simulink model "finalmodel6"  (Simulink 7.5)
settings: Solver=ode23t  StartTime=0.0  StopTime=5  RelTol=1e-3
undefined symbols (not defined in the file): DiscIntNeverNeededParam
libraries: powerlib x5, simulink_extras x3, dspinverses x1, simulink x1
settings Model: Creator=comp  LastModifiedBy=comp

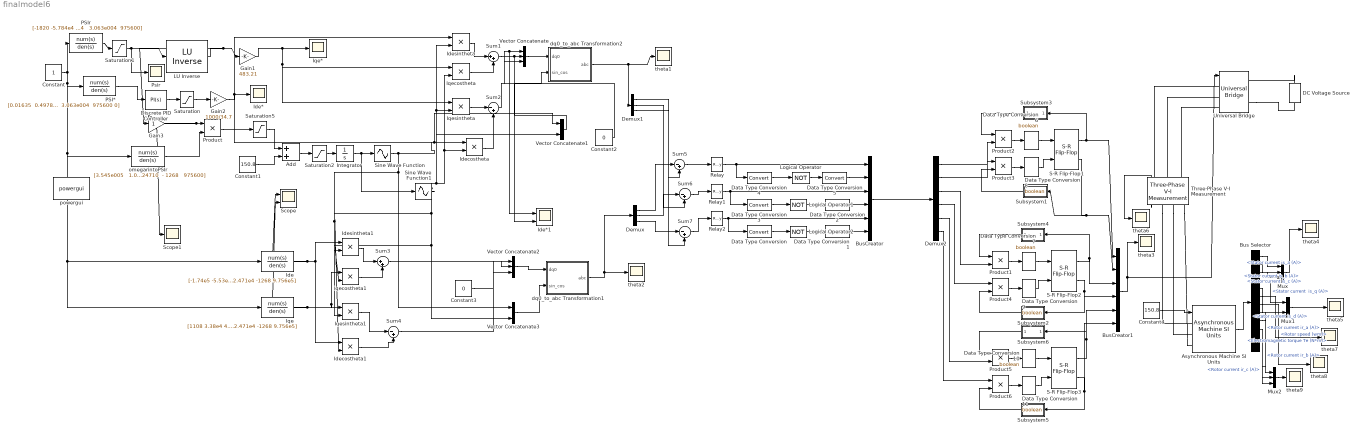
== system finalmodel6 ==
  " LU Inverse" : dspinverses/ LU Inverse  SystemSampleTime=-1
  " omegarintoPSIr" : TransferFcn  Numerator="[3.545e005   1.081e007   1.281e007  - 1.072e010]"  Denominator="[1 - 0.1335  24710  - 1268   975600]"
  Add : Sum  OutDataType=fixdt(1, 16)  OutScaling=2^-10
  Asynchronous Machine SI Units : powerlib/Machines/Asynchronous Machine SI Units  DialogController=POWERSYS.PowerSysDialog  SystemSampleTime=-1  PresetModel=No  MechanicalLoad=Speed w  ShowDetailedParameters=on  RotorType=Squirrel-cage  ReferenceFrame=Stationary  NominalParameters=[149.2e3 400 50]  Stator=[14.85e-3 .3027e-3]  Rotor=[9.295e-3 .3027e-3]  Lm=10.46e-3  Mechanical=[0.0131 0.002985 2]  PolePairs=2  InitialConditions=[1 0 0 0 0 0 0 0]  Units=SI  LoadFlowParameters=1492000  SimulateSaturation=off  Saturation=[14.03593122, 27.81365428, 53.79336849, 72.68890987, 97.98006896, 148.6815601, 215.7428561, 302.9841135, 428.7778367 ; 230, 322, 414, 460, 506, 552, 598, 644, 690]  TsPowergui=0  TsBlock=-1  IterativeModel=Forward Euler
  Bus Selector : BusSelector  OutputSignals="Stator measurements.Stator current is_a (A),Stator measurements.Stator current is_b (A),Stator measurements.Stator current is_c (A),Stator measurements.Stator current  is_q (A),Stator measurements.Stator current is_d (A),Mechanical.Electromagnetic torque Te (N*m),Mechanical.Rotor speed (wm),Rotor measurements.Rotor current ir_a (A),Rotor measurements.Rotor current ir_b (A),Rotor measurements.Rotor current ir_c (A),Rotor measurements.Rotor voltage Vr_q (V),Rotor measurements.Rotor voltage Vr_d (V)"
  BusCreator : BusCreator  Inputs=6
  BusCreator1 : BusCreator  Inputs=6
  Constant : Constant  OutDataType=fixdt(1, 16)  OutScaling=2^0
  Constant1 : Constant  Value=150.8  OutDataType=fixdt(1, 16)  OutScaling=2^0
  Constant2 : Constant  Value=0  OutDataType=fixdt(1, 16)  OutScaling=2^0
  Constant3 : Constant  Value=0  OutDataType=fixdt(1, 16)  OutScaling=2^0
  Constant4 : Constant  Value=150.8  OutDataType=fixdt(1, 16)  OutScaling=2^0
  DC Voltage Source : powerlib/Electrical Sources/DC Voltage Source  DialogController=POWERSYS.PowerSysDialog  SystemSampleTime=-1  Amplitude=400  Measurements=Voltage
  Data Type Conversion{,1..5} (6 alike) : DataTypeConversion  OutDataType=sfix(16)  OutScaling=2^0  SaturateOnIntegerOverflow=on  RndMeth=Zero
  Data Type Conversion{6..11} (6 alike) : DataTypeConversion  OutDataTypeMode=boolean  OutDataType=sfix(16)  OutScaling=2^0  OutDataTypeStr=boolean
  Demux : Demux  Outputs=3
  Demux1 : Demux  Outputs=3
  Demux2 : Demux  Outputs=6
  Discrete PID Controller : simulink/Continuous/PID Controller  DialogController=pidpack.PIDConfig.pidDDGCreate  DialogControllerArgs=DataTag0  SystemSampleTime=-1  Controller=PI  TimeDomain=Continuous-time  SampleTime=1  IntegratorMethod=Forward Euler  FilterMethod=Forward Euler  Form=Parallel  P=100  I=30  D=0  N=100  InitialConditionSource=internal  InitialConditionForIntegrator=0  InitialConditionForFilter=0  ExternalReset=none  LimitOutput=off  UpperSaturationLimit=inf  LowerSaturationLimit=-inf  LinearizeAsGain=off  AntiWindupMode=none  Kb=1  TrackingMode=off  Kt=1  PParamMin=[]  PParamMax=[]  IParamMin=[]  IParamMax=[]  DParamMin=[]  DParamMax=[]  NParamMin=[]  NParamMax=[]  KbParamMin=[]  KbParamMax=[]  KtParamMin=[]  KtParamMax=[]  POutMin=[]  POutMax=[]  IOutMin=[]  IOutMax=[]  DOutMin=[]  DOutMax=[]  NOutMin=[]  NOutMax=[]  KbOutMin=[]  KbOutMax=[]  KtOutMin=[]  KtOutMax=[]  IntegratorOutMin=[]  IntegratorOutMax=[]  FilterOutMin=[]  FilterOutMax=[]  SumOutMin=[]  SumOutMax=[]  SumI1OutMin=[]  SumI1OutMax=[]  SumI2OutMin=[]  SumI2OutMax=[]  SumI3OutMin=[]  SumI3OutMax=[]  SumDOutMin=[]  SumDOutMax=[]  SaturationOutMin=[]  SaturationOutMax=[]  IntegratorContinuousStateAttributes=''  IntegratorStateMustResolveToSignalObject=off  IntegratorRTWStateStorageClass=Auto  FilterContinuousStateAttributes=''  FilterStateMustResolveToSignalObject=off  FilterRTWStateStorageClass=Auto
  Gain1 : Gain  Gain=483.21  ParameterDataType=fixdt(1, 16)  ParameterScaling=2^0  OutDataType=fixdt(1, 16)  OutScaling=2^0  SampleTime=5e-5
  Gain2 : Gain  Gain=1000/34.7  ParameterDataType=fixdt(1, 16)  ParameterScaling=2^0  OutDataType=fixdt(1, 16)  OutScaling=2^0  SampleTime=5e-5
  Gain3 : Gain  ParameterDataType=fixdt(1, 16)  ParameterScaling=2^0  OutDataType=fixdt(1, 16)  OutScaling=2^0  SampleTime=5e-5
  Ide : TransferFcn  Numerator=[-1.74e5 -5.53e6 -6.725e6]  Denominator=[1 -.1335 2.471e4 -1268 9.756e5]
  Ide* : Scope
      settings: YMin=-100  YMax=100
  Ide*1 : Scope  NumInputPorts=2
      settings: YMin=-10000~-1000  YMax=10000~1000  SaveName=ScopeData5
  Idecostheta : Product  OutDataType=fixdt(1, 16)  OutScaling=2^0  RndMeth=Zero
  Idecostheta1 : Product  OutDataType=fixdt(1, 16)  OutScaling=2^0  RndMeth=Zero
  Idesintheta : Product  OutDataType=fixdt(1, 16)  OutScaling=2^0  RndMeth=Zero
  Idesintheta1 : Product  OutDataType=fixdt(1, 16)  OutScaling=2^0  RndMeth=Zero
  Integrator : Integrator  UpperSaturationLimit=pi/5  LowerSaturationLimit=0
  Iqe : TransferFcn  Numerator=[1108 3.38e4 4.003e4 -3.349e7]  Denominator=[1 -.1335 2.471e4 -1268 9.756e5]
  Iqe* : Scope
      settings: YMin=-200  YMax=200
  Iqecostheta : Product  OutDataType=fixdt(1, 16)  OutScaling=2^0  RndMeth=Zero
  Iqecostheta1 : Product  OutDataType=fixdt(1, 16)  OutScaling=2^0  RndMeth=Zero
  Iqesintheta : Product  OutDataType=fixdt(1, 16)  OutScaling=2^0  RndMeth=Zero
  Iqesintheta1 : Product  OutDataType=fixdt(1, 16)  OutScaling=2^0  RndMeth=Zero
  Logical Operator : Logic  Operator=NOT
  Logical Operator1 : Logic  Operator=NOT
  Logical Operator2 : Logic  Operator=NOT
  Mux : Mux  Inputs=3
  Mux1 : Mux  Inputs=2
  Mux2 : Mux  Inputs=3
  PSI* : TransferFcn  Numerator="[0.01635  0.4978 2224  7.018e004  8.566e004   487800]"  Denominator="[0.03269 0.9956  807.7  2.467e004  3.063e004  975600 0]"
  PSIr : TransferFcn  Numerator=[-1820 -5.784e4 -7.034e4]  Denominator="[0.03269   0.9956   807.7   2.467e004   3.063e004  975600]"
  Product : Product  OutDataType=fixdt(1, 16)  OutScaling=2^0  RndMeth=Zero
  Product{1..6} (6 alike) : Product  OutDataType=sfix(16)  OutScaling=2^0  RndMeth=Zero
  Psir : Scope
      settings: YMin=-10  YMax=10  SaveName=ScopeData4
  Relay : Relay  OnSwitchValue=5  OffSwitchValue=-5  OutDataType=sfix(16)  OutScaling=2^0
  Relay1 : Relay  OnSwitchValue=5  OffSwitchValue=-5  OutDataType=sfix(16)  OutScaling=2^0
  Relay2 : Relay  OnSwitchValue=5  OffSwitchValue=-5  OutDataType=sfix(16)  OutScaling=2^0
  S-R Flip-Flop1 : simulink_extras/Flip Flops/S-R Flip-Flop  SystemSampleTime=-1  initial_condition=0
  S-R Flip-Flop2 : simulink_extras/Flip Flops/S-R Flip-Flop  SystemSampleTime=-1  initial_condition=0
  S-R Flip-Flop3 : simulink_extras/Flip Flops/S-R Flip-Flop  SystemSampleTime=-1  initial_condition=0
  Saturation : Saturate  UpperLimit=2  LowerLimit=-2
  Saturation1 : Saturate  UpperLimit=-.7  LowerLimit=-.7
  Saturation2 : Saturate  UpperLimit=170  LowerLimit=-130
  Saturation5 : Saturate  UpperLimit=7.08  LowerLimit=-7.08
  Scope : Scope  NumInputPorts=2
      settings: YMin=-5~-5  YMax=5~5  SaveName=ScopeData12
  Scope1 : Scope
      settings: YMin=-100  YMax=100  SaveName=ScopeData13
  Sine Wave Function : Sin  TimeSource=Use external signal  Amplitude=1  Bias=0  Frequency=1  Phase=0  Samples=10  SampleTime=0  Offset=0
  Sine Wave Function1 : Sin  TimeSource=Use external signal  Amplitude=1  Bias=0  Frequency=1  Phase=+pi/2  Samples=10  SampleTime=0  Offset=0
  Subsystem1 : Subsystem
  Subsystem2 : Subsystem
  Subsystem3 : Subsystem
  Subsystem4 : Subsystem
  Subsystem5 : Subsystem
  Subsystem6 : Subsystem
  Sum1 : Sum  Inputs=|++  OutDataType=fixdt(1, 16)  OutScaling=2^0
  Sum{2,4..7} (5 alike) : Sum  Inputs=|-+  OutDataType=fixdt(1, 16)  OutScaling=2^0
  Sum3 : Sum  Inputs=|++  OutDataType=fixdt(1, 16)  OutScaling=2^0
  Three-Phase V-I Measurement : powerlib/Measurements/Three-Phase V-I Measurement  DialogController=POWERSYS.PowerSysDialog  SystemSampleTime=-1  VoltageMeasurement=phase-to-phase  SetLabelV=off  LabelV=Vabc  Vpu=off  VpuLL=off  CurrentMeasurement=no  SetLabelI=off  LabelI=Iabc  Ipu=off  Pbase=100e6  Vbase=500e3  OutputType=Complex  PhasorSimulation=off  PSBequivalent=0
  Universal Bridge : powerlib/Power Electronics/Universal Bridge  DialogController=POWERSYS.PowerSysDialog  SystemSampleTime=-1  Arms=3  SnubberResistance=5e3  SnubberCapacitance=inf  Device=IGBT / Diodes  Ron=1e-3  Lon=0  ForwardVoltages=[.8,.8]  ForwardVoltage=0  GTOparameters=[ 10e-6 , 20e-6 ]  IGBTparameters=[ 1e-6 , 2e-6 ]  Measurements=All voltages and currents  Measurements_2=None  converterType=Rectifier
  Vector Concatenate : Concatenate  NumInputs=3  Mode=Vector
  Vector Concatenate1 : Concatenate  Mode=Vector
  Vector Concatenate2 : Concatenate  NumInputs=3  Mode=Vector
  Vector Concatenate3 : Concatenate  Mode=Vector
  dq0_to_abc Transformation1 : Subsystem  AncestorBlock=powerlib_extras/Measurements/dq0_to_abc Transformation  DialogController=POWERSYS.PowerSysDialog  mask(dq0 to abc Transformation){}
      mask help:
      | This block transforms  three quantities  (direct axis, quadature axis and zero-sequence components)  expressed in a two axis reference frame back to phase quantities.
      |
      | The following transformation is used:
      |
      | Va = [Vd*sin(wt) +  Vq*cos(wt)  +  Vo ]
      | Vb = [Vd*sin(wt-2pi/3)  + Vq*cos(wt-2pi/3)  + Vo)
      | Vc = [Vd*sin(wt+2pi/3) + Vq*cos(wt+2pi/3)  + Vo)
      | where w=  rotation speed (rad/s) of the rotating frame.
      |
      | Input 1 contains  the vectorized signal of [Vd Vq  Vo] components
      | Input 2 must contain a  [sin(wt)  cos(wt)] two dimension signal , where w is the rotation speed  of the reference frame.
      | Output is a vectozized signal containing the three  [Va Vb Vc] phase sinusoidal quantities.
      |
      | Press Help for more information.
      mask init:
      | power_initmask();
      mask Help: web(psbhelp)
      mask Display: disp('')
  dq0_to_abc Transformation2 : Subsystem  AncestorBlock=powerlib_extras/Measurements/dq0_to_abc Transformation  DialogController=POWERSYS.PowerSysDialog  mask(dq0 to abc Transformation){}
      mask help:
      | This block transforms  three quantities  (direct axis, quadature axis and zero-sequence components)  expressed in a two axis reference frame back to phase quantities.
      |
      | The following transformation is used:
      |
      | Va = [Vd*sin(wt) +  Vq*cos(wt)  +  Vo ]
      | Vb = [Vd*sin(wt-2pi/3)  + Vq*cos(wt-2pi/3)  + Vo)
      | Vc = [Vd*sin(wt+2pi/3) + Vq*cos(wt+2pi/3)  + Vo)
      | where w=  rotation speed (rad/s) of the rotating frame.
      |
      | Input 1 contains  the vectorized signal of [Vd Vq  Vo] components
      | Input 2 must contain a  [sin(wt)  cos(wt)] two dimension signal , where w is the rotation speed  of the reference frame.
      | Output is a vectozized signal containing the three  [Va Vb Vc] phase sinusoidal quantities.
      |
      | Press Help for more information.
      mask init:
      | power_initmask();
      mask Help: web(psbhelp)
      mask Display: disp('')
  powergui : powerlib/powergui  Priority=1  SystemSampleTime=-1  SimulationMode=Discrete  SampleTime=50e-6  frequency=60  SPID=off  DisableSnubberDevices=off  DisableRonSwitches=off  DisableVfSwitches=off  SwTol=0  Interpol=off  frequencyindice=50  echomessages=off  HookPort=off  DisplayEquations=off  FunctionMessages=off  EnableUseOfTLC=off  x0status=blocks  RestoreLinks=warning  ResistiveCurrentMeasurement=off  Ylog=off  Xlog=on  ShowGrid=off  save=off  variable=ZData  ZoomFFT=off  StartTime=0.0  cycles=1  DisplayStyle=1  FreqAxis=off  MaxFrequency=1000  frequencyindicesteady=1  display=off  methode=off
  theta{1..9} (9 alike) : Scope
      theta1 settings: YMin=-90  YMax=90  SaveName=ScopeData3
      theta2 settings: TimeRange=5  YMin=-800  YMax=800  SaveName=ScopeData2
      theta3 settings: TimeRange=10  YMin=0  YMax=1  SaveName=ScopeData6
      theta4 settings: TimeRange=10  YMin=-1500  YMax=1500  SaveName=ScopeData7
      theta5 settings: TimeRange=10  YMin=-1500  YMax=1500  SaveName=ScopeData8
      theta6 settings: TimeRange=5  YMin=-1  YMax=1  SaveName=ScopeData9
      theta7 settings: TimeRange=5  YMin=1525  YMax=1875  SaveName=ScopeData10
      theta8 settings: TimeRange=10  YMin=143.26  YMax=158.34  SaveName=ScopeData11
      theta9 settings: TimeRange=10  YMin=-1250  YMax=1500  SaveName=ScopeData14
  wires:
  Constant/1 -> PSIr/1, PSI*/1, " omegarintoPSIr"/1, Ide/1, Iqe/1
  PSIr/1 -> Saturation1/1
  " LU Inverse"/1 -> Gain1/1, Gain3/1
  Gain1/1 -> Iqe*/1, Iqecostheta/1, Iqesintheta/1
  PSI*/1 -> Discrete PID Controller/1
  Gain2/1 -> Ide*/1, Idesintheta/1, Idecostheta/1
  " omegarintoPSIr"/1 -> Product/2
  Constant1/1 -> Add/2
  Idecostheta/1 -> Sum2/2
  Iqesintheta/1 -> Sum2/1
  Idesintheta/1 -> Sum1/1
  Iqecostheta/1 -> Sum1/2
  Sine Wave Function1/1 -> Idecostheta/2, Iqecostheta/2, Vector Concatenate1/2, Idecostheta1/2, Vector Concatenate3/2, Iqecostheta1/2
  Sum1/1 -> Vector Concatenate/2, Ide*1/2
  Sum2/1 -> Vector Concatenate/1, Ide*1/1
  Constant2/1 -> Vector Concatenate/3
  Vector Concatenate/1 -> dq0_to_abc Transformation2/1(dq0)
  Vector Concatenate1/1 -> dq0_to_abc Transformation2/2(sin_cos)
  Product/1 -> Saturation5/1
  Integrator/1 -> Sine Wave Function/1, Sine Wave Function1/1
  Sine Wave Function/1 -> Idesintheta/2, Iqesintheta/2, Vector Concatenate1/1, Vector Concatenate3/1, Idesintheta1/2, Iqesintheta1/2
  Vector Concatenate2/1 -> dq0_to_abc Transformation1/1(dq0)
  Vector Concatenate3/1 -> dq0_to_abc Transformation1/2(sin_cos)
  Idesintheta1/1 -> Sum3/1
  Iqecostheta1/1 -> Sum3/2
  Iqesintheta1/1 -> Sum4/1
  Idecostheta1/1 -> Sum4/2
  Sum3/1 -> Vector Concatenate2/2
  Constant3/1 -> Vector Concatenate2/3
  Ide/1 -> Idesintheta1/1, Idecostheta1/1, Scope/1
  Iqe/1 -> Iqecostheta1/1, Iqesintheta1/1, Scope/2
  dq0_to_abc Transformation1/1(abc) -> theta2/1, Demux/1
  Demux/1 -> Sum5/1
  Demux/2 -> Sum6/1
  Demux/3 -> Sum7/1
  Demux1/1 -> Sum5/2
  Demux1/3 -> Sum7/2
  Gain3/1 -> Product/1, Scope1/1
  Saturation/1 -> Gain2/1
  Discrete PID Controller/1 -> Saturation/1
  Saturation1/1 -> " LU Inverse"/1, Psir/1
  Add/1 -> Saturation2/1
  Saturation2/1 -> Integrator/1
  dq0_to_abc Transformation2/1(abc) -> theta1/1, Demux1/1
  Logical Operator2/1 -> Data Type Conversion1/1
  Logical Operator1/1 -> Data Type Conversion2/1
  Logical Operator/1 -> Data Type Conversion5/1
  Relay2/1 -> BusCreator/5, Data Type Conversion/1
  Relay1/1 -> BusCreator/3, Data Type Conversion3/1
  Relay/1 -> BusCreator/1, Data Type Conversion4/1
  Data Type Conversion/1 -> Logical Operator2/1
  Data Type Conversion1/1 -> BusCreator/6
  Data Type Conversion2/1 -> BusCreator/4
  Data Type Conversion3/1 -> Logical Operator1/1
  Data Type Conversion4/1 -> Logical Operator/1
  Data Type Conversion5/1 -> BusCreator/2
  Demux1/2 -> Sum6/2
  Sum5/1 -> Relay/1
  Sum6/1 -> Relay1/1
  Sum7/1 -> Relay2/1
  Demux2/2 -> Product3/1
  Demux2/1 -> Product2/2
  Subsystem1/1(Trig) -> Product3/2
  S-R Flip-Flop1/2 -> Subsystem1/1(Sig), BusCreator1/2
  Product3/1 -> Data Type Conversion8/1
  Data Type Conversion8/1 -> S-R Flip-Flop1/2
  Data Type Conversion6/1 -> S-R Flip-Flop1/1
  Subsystem3/1(Trig) -> Product2/1
  Product2/1 -> Data Type Conversion6/1
  S-R Flip-Flop1/1 -> BusCreator1/1, Subsystem3/1(Sig)
  BusCreator/1 -> Demux2/1
  Subsystem2/1(Trig) -> Product4/2
  S-R Flip-Flop2/2 -> Subsystem2/1(Sig), BusCreator1/4
  Product4/1 -> Data Type Conversion9/1
  Data Type Conversion9/1 -> S-R Flip-Flop2/2
  Data Type Conversion7/1 -> S-R Flip-Flop2/1
  Subsystem4/1(Trig) -> Product1/1
  Product1/1 -> Data Type Conversion7/1
  Demux2/3 -> Product1/2
  Demux2/4 -> Product4/1
  Subsystem5/1(Trig) -> Product6/2
  S-R Flip-Flop3/2 -> Subsystem5/1(Sig), BusCreator1/6
  Product6/1 -> Data Type Conversion11/1
  Data Type Conversion11/1 -> S-R Flip-Flop3/2
  Data Type Conversion10/1 -> S-R Flip-Flop3/1
  Subsystem6/1(Trig) -> Product5/1
  Product5/1 -> Data Type Conversion10/1
  S-R Flip-Flop3/1 -> Subsystem6/1(Sig), BusCreator1/5
  Demux2/5 -> Product5/2
  Demux2/6 -> Product6/1
  S-R Flip-Flop2/1 -> Subsystem4/1(Sig), BusCreator1/3
  BusCreator1/1 -> theta3/1, Universal Bridge/1
  Asynchronous Machine SI Units/1 -> Bus Selector/1
  Bus Selector/1 -> Mux/1  "<Stator current is_a (A)>"
  Bus Selector/2 -> Mux/2  "<Stator current is_b (A)>"
  Bus Selector/3 -> Mux/3  "<Stator current is_c (A)>"
  Mux/1 -> theta4/1
  Bus Selector/4 -> Mux1/1  "<Stator current  is_q (A)>"
  Bus Selector/5 -> Mux1/2  "<Stator current is_d (A)>"
  Mux1/1 -> theta5/1
  Three-Phase V-I Measurement/1 -> theta6/1
  Bus Selector/7 -> theta8/1  "<Rotor speed (wm)>"
  Bus Selector/6 -> theta7/1  "<Electromagnetic torque Te (N*m)>"
  Saturation5/1 -> Add/1
  Mux2/1 -> theta9/1
  Bus Selector/8 -> Mux2/1  "<Rotor current ir_a (A)>"
  Bus Selector/9 -> Mux2/2  "<Rotor current ir_b (A)>"
  Bus Selector/10 -> Mux2/3  "<Rotor current ir_c (A)>"
  Constant4/1 -> Asynchronous Machine SI Units/1
  Sum4/1 -> Vector Concatenate2/1
  connections:
  DC Voltage Source/RConn1 -- Universal Bridge/RConn1
  Universal Bridge/RConn2 -- DC Voltage Source/LConn1
  Three-Phase V-I Measurement/RConn3 -- Asynchronous Machine SI Units/LConn3
  Three-Phase V-I Measurement/RConn2 -- Asynchronous Machine SI Units/LConn2
  Three-Phase V-I Measurement/RConn1 -- Asynchronous Machine SI Units/LConn1
  Universal Bridge/LConn3 -- Three-Phase V-I Measurement/LConn3
  Universal Bridge/LConn2 -- Three-Phase V-I Measurement/LConn2
  Universal Bridge/LConn1 -- Three-Phase V-I Measurement/LConn1

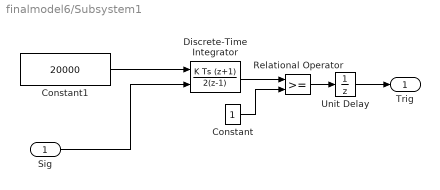
== system finalmodel6/Subsystem1 ==
  Sig : Inport  OutDataType=sfix(16)  OutScaling=2^0
  Constant : Constant  OutDataType=sfix(16)  OutScaling=2^0
  Constant1 : Constant  Value=20000  OutDataType=sfix(16)  OutScaling=2^0
  Discrete-Time Integrator : DiscreteIntegrator  IntegratorMethod=Integration: Trapezoidal  ExternalReset=rising  SampleTime=5e-5  OutDataType=sfix(16)  OutScaling=2^0  ICPrevOutput=DiscIntNeverNeededParam  ICPrevScaledInput=DiscIntNeverNeededParam
  Relational Operator : RelationalOperator  ZeroCross=off
  Unit Delay : UnitDelay  SampleTime=-1
  Trig : Outport  OutDataType=sfix(16)  OutScaling=2^0
  wires:
  Unit Delay/1 -> Trig/1
  Sig/1 -> Discrete-Time Integrator/2
  Relational Operator/1 -> Unit Delay/1
  Discrete-Time Integrator/1 -> Relational Operator/1
  Constant/1 -> Relational Operator/2
  Constant1/1 -> Discrete-Time Integrator/1

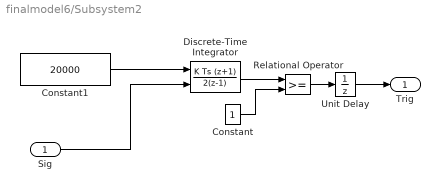
== system finalmodel6/Subsystem2 ==
  Sig : Inport  OutDataType=sfix(16)  OutScaling=2^0
  Constant : Constant  OutDataType=sfix(16)  OutScaling=2^0
  Constant1 : Constant  Value=20000  OutDataType=sfix(16)  OutScaling=2^0
  Discrete-Time Integrator : DiscreteIntegrator  IntegratorMethod=Integration: Trapezoidal  ExternalReset=rising  SampleTime=5e-5  OutDataType=sfix(16)  OutScaling=2^0  ICPrevOutput=DiscIntNeverNeededParam  ICPrevScaledInput=DiscIntNeverNeededParam
  Relational Operator : RelationalOperator  ZeroCross=off
  Unit Delay : UnitDelay  SampleTime=-1
  Trig : Outport  OutDataType=sfix(16)  OutScaling=2^0
  wires:
  Unit Delay/1 -> Trig/1
  Sig/1 -> Discrete-Time Integrator/2
  Relational Operator/1 -> Unit Delay/1
  Discrete-Time Integrator/1 -> Relational Operator/1
  Constant/1 -> Relational Operator/2
  Constant1/1 -> Discrete-Time Integrator/1

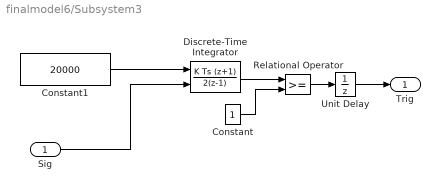
== system finalmodel6/Subsystem3 ==
  Sig : Inport  OutDataType=sfix(16)  OutScaling=2^0
  Constant : Constant  OutDataType=sfix(16)  OutScaling=2^0
  Constant1 : Constant  Value=20000  OutDataType=sfix(16)  OutScaling=2^0
  Discrete-Time Integrator : DiscreteIntegrator  IntegratorMethod=Integration: Trapezoidal  ExternalReset=rising  SampleTime=5e-5  OutDataType=sfix(16)  OutScaling=2^0  ICPrevOutput=DiscIntNeverNeededParam  ICPrevScaledInput=DiscIntNeverNeededParam
  Relational Operator : RelationalOperator  ZeroCross=off
  Unit Delay : UnitDelay  SampleTime=-1
  Trig : Outport  OutDataType=sfix(16)  OutScaling=2^0
  wires:
  Constant1/1 -> Discrete-Time Integrator/1
  Constant/1 -> Relational Operator/2
  Discrete-Time Integrator/1 -> Relational Operator/1
  Relational Operator/1 -> Unit Delay/1
  Sig/1 -> Discrete-Time Integrator/2
  Unit Delay/1 -> Trig/1

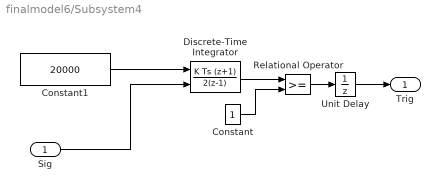
== system finalmodel6/Subsystem4 ==
  Sig : Inport  OutDataType=sfix(16)  OutScaling=2^0
  Constant : Constant  OutDataType=sfix(16)  OutScaling=2^0
  Constant1 : Constant  Value=20000  OutDataType=sfix(16)  OutScaling=2^0
  Discrete-Time Integrator : DiscreteIntegrator  IntegratorMethod=Integration: Trapezoidal  ExternalReset=rising  SampleTime=5e-5  OutDataType=sfix(16)  OutScaling=2^0  ICPrevOutput=DiscIntNeverNeededParam  ICPrevScaledInput=DiscIntNeverNeededParam
  Relational Operator : RelationalOperator  ZeroCross=off
  Unit Delay : UnitDelay  SampleTime=-1
  Trig : Outport  OutDataType=sfix(16)  OutScaling=2^0
  wires:
  Constant1/1 -> Discrete-Time Integrator/1
  Constant/1 -> Relational Operator/2
  Discrete-Time Integrator/1 -> Relational Operator/1
  Relational Operator/1 -> Unit Delay/1
  Sig/1 -> Discrete-Time Integrator/2
  Unit Delay/1 -> Trig/1

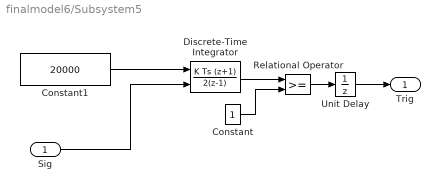
== system finalmodel6/Subsystem5 ==
  Sig : Inport  OutDataType=sfix(16)  OutScaling=2^0
  Constant : Constant  OutDataType=sfix(16)  OutScaling=2^0
  Constant1 : Constant  Value=20000  OutDataType=sfix(16)  OutScaling=2^0
  Discrete-Time Integrator : DiscreteIntegrator  IntegratorMethod=Integration: Trapezoidal  ExternalReset=rising  SampleTime=5e-5  OutDataType=sfix(16)  OutScaling=2^0  ICPrevOutput=DiscIntNeverNeededParam  ICPrevScaledInput=DiscIntNeverNeededParam
  Relational Operator : RelationalOperator  ZeroCross=off
  Unit Delay : UnitDelay  SampleTime=-1
  Trig : Outport  OutDataType=sfix(16)  OutScaling=2^0
  wires:
  Unit Delay/1 -> Trig/1
  Sig/1 -> Discrete-Time Integrator/2
  Relational Operator/1 -> Unit Delay/1
  Discrete-Time Integrator/1 -> Relational Operator/1
  Constant/1 -> Relational Operator/2
  Constant1/1 -> Discrete-Time Integrator/1

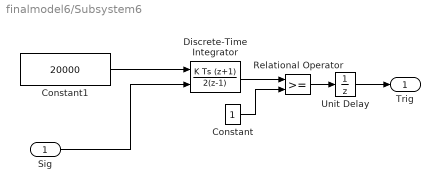
== system finalmodel6/Subsystem6 ==
  Sig : Inport  OutDataType=sfix(16)  OutScaling=2^0
  Constant : Constant  OutDataType=sfix(16)  OutScaling=2^0
  Constant1 : Constant  Value=20000  OutDataType=sfix(16)  OutScaling=2^0
  Discrete-Time Integrator : DiscreteIntegrator  IntegratorMethod=Integration: Trapezoidal  ExternalReset=rising  SampleTime=5e-5  OutDataType=sfix(16)  OutScaling=2^0  ICPrevOutput=DiscIntNeverNeededParam  ICPrevScaledInput=DiscIntNeverNeededParam
  Relational Operator : RelationalOperator  ZeroCross=off
  Unit Delay : UnitDelay  SampleTime=-1
  Trig : Outport  OutDataType=sfix(16)  OutScaling=2^0
  wires:
  Constant1/1 -> Discrete-Time Integrator/1
  Constant/1 -> Relational Operator/2
  Discrete-Time Integrator/1 -> Relational Operator/1
  Relational Operator/1 -> Unit Delay/1
  Sig/1 -> Discrete-Time Integrator/2
  Unit Delay/1 -> Trig/1

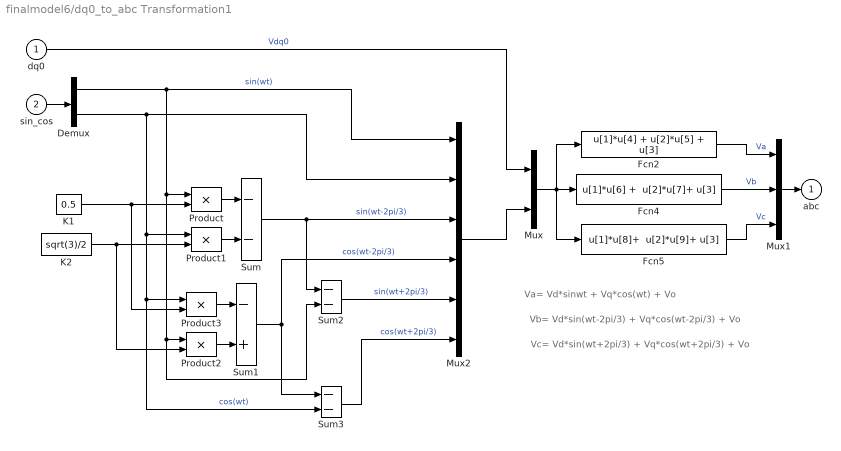
== system finalmodel6/dq0_to_abc Transformation1 ==
  note: Vc= Vd*sin(wt+2pi/3) + Vq*cos(wt+2pi/3) + Vo
  note: Vb= Vd*sin(wt-2pi/3) + Vq*cos(wt-2pi/3) + Vo
  note: Va= Vd*sinwt + Vq*cos(wt) + Vo
  dq0 : Inport  PortDimensions=3  OutDataType=sfix(16)  OutScaling=2^0
  sin_cos : Inport  Port=2  PortDimensions=2  OutDataType=sfix(16)  OutScaling=2^0
  Demux : Demux  Outputs=2
  Fcn2 : Fcn  Expr="u[1]*u[4] +  u[2]*u[5] + u[3]"
  Fcn4 : Fcn  Expr="u[1]*u[6] +  u[2]*u[7]+ u[3]"
  Fcn5 : Fcn  Expr="u[1]*u[8]+  u[2]*u[9]+ u[3]"
  K1 : Constant  Value=0.5  OutDataType=sfix(16)  OutScaling=2^0
  K2 : Constant  Value=sqrt(3)/2  OutDataType=sfix(16)  OutScaling=2^0
  Mux : Mux  Inputs=2
  Mux1 : Mux  Inputs=3
  Mux2 : Mux  Inputs=6
  Product{,1..3} (4 alike) : Product  OutDataType=sfix(16)  OutScaling=2^0  SaturateOnIntegerOverflow=on  InputSameDT=on  OutDataTypeStr=Inherit: Same as first input
  Sum : Sum  Inputs=--  OutDataType=sfix(16)  OutScaling=2^0  SaturateOnIntegerOverflow=on  InputSameDT=on  OutDataTypeStr=Inherit: Same as first input
  Sum1 : Sum  Inputs=-+  OutDataType=sfix(16)  OutScaling=2^0  SaturateOnIntegerOverflow=on  InputSameDT=on  OutDataTypeStr=Inherit: Same as first input
  Sum2 : Sum  Inputs=--  OutDataType=sfix(16)  OutScaling=2^0  SaturateOnIntegerOverflow=on  InputSameDT=on  OutDataTypeStr=Inherit: Same as first input
  Sum3 : Sum  Inputs=--  OutDataType=sfix(16)  OutScaling=2^0  SaturateOnIntegerOverflow=on  InputSameDT=on  OutDataTypeStr=Inherit: Same as first input
  abc : Outport  OutDataType=sfix(16)  OutScaling=2^0  InitialOutput=0
  wires:
  dq0/1 -> Mux/1  "Vdq0"
  Mux2/1 -> Mux/2
  sin_cos/1 -> Demux/1
  Demux/2 -> Sum3/2, Product3/1, Product1/1, Mux2/2  "cos(wt)"
  Demux/1 -> Product/1, Product2/1, Sum2/2, Mux2/1  "sin(wt)"
  Product/1 -> Sum/1
  Product1/1 -> Sum/2
  Product3/1 -> Sum1/1
  Product2/1 -> Sum1/2
  Sum3/1 -> Mux2/6  "cos(wt+2pi/3)"
  Sum2/1 -> Mux2/5  "sin(wt+2pi/3)"
  K1/1 -> Product/2, Product3/2
  K2/1 -> Product1/2, Product2/2
  Sum/1 -> Mux2/3, Sum2/1  "sin(wt-2pi/3)"
  Sum1/1 -> Mux2/4, Sum3/1  "cos(wt-2pi/3)"
  Mux/1 -> Fcn5/1, Fcn2/1, Fcn4/1
  Mux1/1 -> abc/1
  Fcn2/1 -> Mux1/1  "Va"
  Fcn4/1 -> Mux1/2  "Vb"
  Fcn5/1 -> Mux1/3  "Vc"

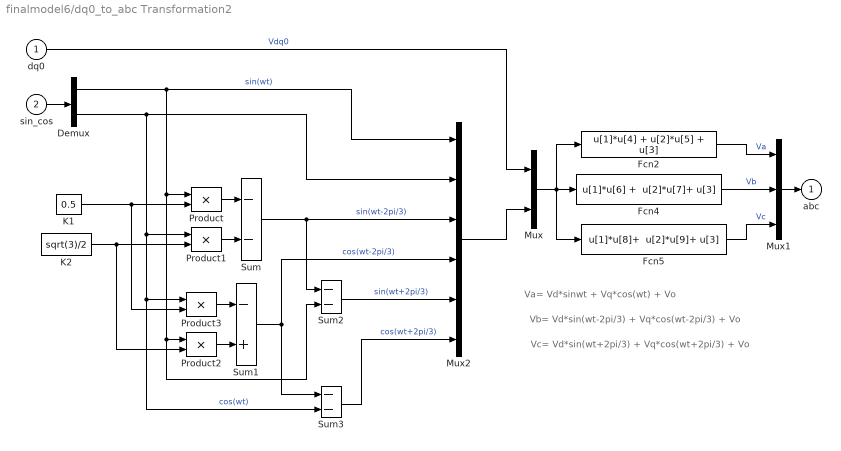
== system finalmodel6/dq0_to_abc Transformation2 ==
  note: Vc= Vd*sin(wt+2pi/3) + Vq*cos(wt+2pi/3) + Vo
  note: Vb= Vd*sin(wt-2pi/3) + Vq*cos(wt-2pi/3) + Vo
  note: Va= Vd*sinwt + Vq*cos(wt) + Vo
  dq0 : Inport  PortDimensions=3  OutDataType=sfix(16)  OutScaling=2^0
  sin_cos : Inport  Port=2  PortDimensions=2  OutDataType=sfix(16)  OutScaling=2^0
  Demux : Demux  Outputs=2
  Fcn2 : Fcn  Expr="u[1]*u[4] +  u[2]*u[5] + u[3]"
  Fcn4 : Fcn  Expr="u[1]*u[6] +  u[2]*u[7]+ u[3]"
  Fcn5 : Fcn  Expr="u[1]*u[8]+  u[2]*u[9]+ u[3]"
  K1 : Constant  Value=0.5  OutDataType=sfix(16)  OutScaling=2^0
  K2 : Constant  Value=sqrt(3)/2  OutDataType=sfix(16)  OutScaling=2^0
  Mux : Mux  Inputs=2
  Mux1 : Mux  Inputs=3
  Mux2 : Mux  Inputs=6
  Product{,1..3} (4 alike) : Product  OutDataType=sfix(16)  OutScaling=2^0  SaturateOnIntegerOverflow=on  InputSameDT=on  OutDataTypeStr=Inherit: Same as first input
  Sum : Sum  Inputs=--  OutDataType=sfix(16)  OutScaling=2^0  SaturateOnIntegerOverflow=on  InputSameDT=on  OutDataTypeStr=Inherit: Same as first input
  Sum1 : Sum  Inputs=-+  OutDataType=sfix(16)  OutScaling=2^0  SaturateOnIntegerOverflow=on  InputSameDT=on  OutDataTypeStr=Inherit: Same as first input
  Sum2 : Sum  Inputs=--  OutDataType=sfix(16)  OutScaling=2^0  SaturateOnIntegerOverflow=on  InputSameDT=on  OutDataTypeStr=Inherit: Same as first input
  Sum3 : Sum  Inputs=--  OutDataType=sfix(16)  OutScaling=2^0  SaturateOnIntegerOverflow=on  InputSameDT=on  OutDataTypeStr=Inherit: Same as first input
  abc : Outport  OutDataType=sfix(16)  OutScaling=2^0  InitialOutput=0
  wires:
  dq0/1 -> Mux/1  "Vdq0"
  Mux2/1 -> Mux/2
  sin_cos/1 -> Demux/1
  Demux/2 -> Sum3/2, Product3/1, Product1/1, Mux2/2  "cos(wt)"
  Demux/1 -> Product/1, Product2/1, Sum2/2, Mux2/1  "sin(wt)"
  Product/1 -> Sum/1
  Product1/1 -> Sum/2
  Product3/1 -> Sum1/1
  Product2/1 -> Sum1/2
  Sum3/1 -> Mux2/6  "cos(wt+2pi/3)"
  Sum2/1 -> Mux2/5  "sin(wt+2pi/3)"
  K1/1 -> Product/2, Product3/2
  K2/1 -> Product1/2, Product2/2
  Sum/1 -> Mux2/3, Sum2/1  "sin(wt-2pi/3)"
  Sum1/1 -> Mux2/4, Sum3/1  "cos(wt-2pi/3)"
  Mux/1 -> Fcn5/1, Fcn2/1, Fcn4/1
  Mux1/1 -> abc/1
  Fcn2/1 -> Mux1/1  "Va"
  Fcn4/1 -> Mux1/2  "Vb"
  Fcn5/1 -> Mux1/3  "Vc"
